simulink model "radar2jammer_god"  (R2024a)
settings: Solver=VariableStepAuto  StartTime=0.0  StopTime=inf  RelTol=1e-3
libraries: robotlib x6
settings Model: PacingRate=0.890000  Creator=bitdol  LastModifiedBy=user

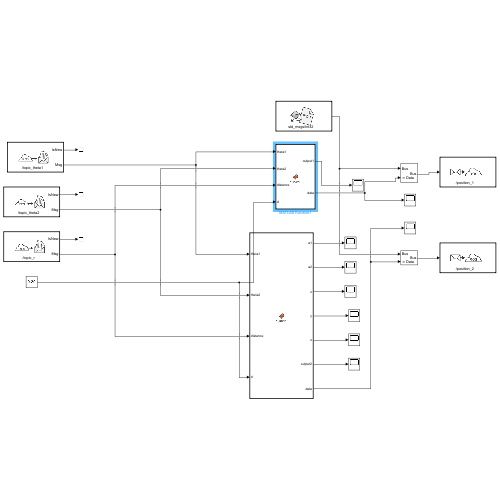
[thumbnail: Simulink's stored preview of the top-level diagram]
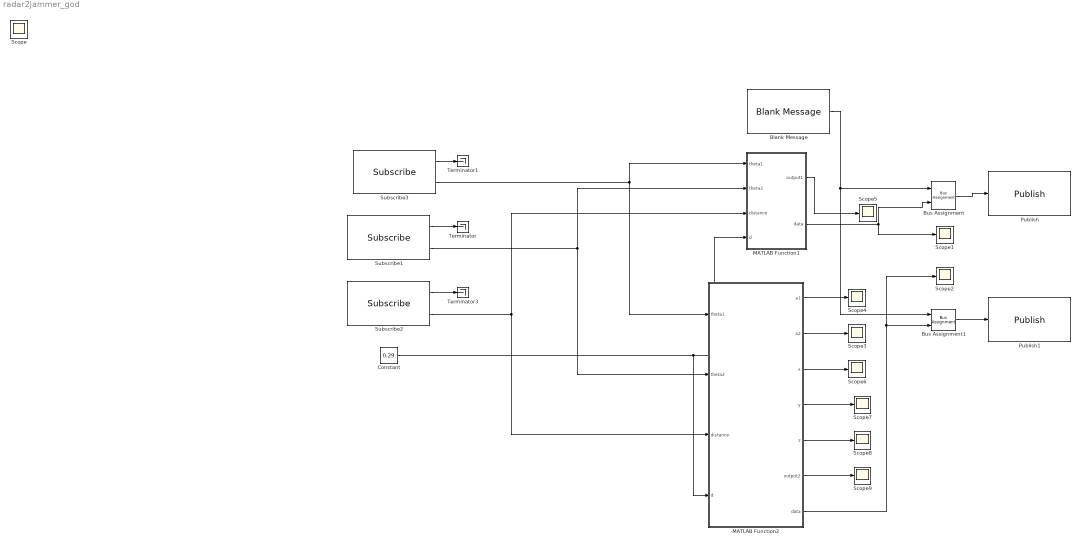
== system radar2jammer_god ==
  Blank Message : robotlib/Blank Message  messageClass=Message  entityType=std_msgs/Int32  messageType=std_msgs/Int32  SampleTime=inf  legacyBusStruct=off
  Bus Assignment : BusAssignment  AssignedSignals=Data
  Bus Assignment1 : BusAssignment  AssignedSignals=Data
  Constant : Constant  Value=0.29
  MATLAB Function1 : MATLAB Function  TreatAsAtomicUnit=on
  MATLAB Function2 : MATLAB Function  TreatAsAtomicUnit=on
  Publish : robotlib/Publish  topicSource=Specify your own  topic=/position_1  messageType=std_msgs/Int32  legacyBusStruct=off  messageQueueLength=1
  Publish1 : robotlib/Publish  topicSource=Specify your own  topic=/position_2  messageType=std_msgs/Int32  legacyBusStruct=off  messageQueueLength=1
  Scope{,1..9} (10 alike) : Scope
  Subscribe1 : robotlib/Subscribe  topicSource=Select from ROS network  topic=/topic_theta2  messageType=std_msgs/Int32  SampleTime=-1  legacyBusStruct=off  messageQueueLength=1
  Subscribe2 : robotlib/Subscribe  topicSource=Select from ROS network  topic=/topic_r  messageType=std_msgs/Int32  SampleTime=-1  legacyBusStruct=off  messageQueueLength=1
  Subscribe3 : robotlib/Subscribe  topicSource=Select from ROS network  topic=/topic_theta1  messageType=std_msgs/Int32  SampleTime=-1  legacyBusStruct=off  messageQueueLength=1
  Terminator : Terminator
  Terminator1 : Terminator
  Terminator3 : Terminator
  wires:
  Subscribe2/1 -> Terminator3/1
  Subscribe3/1 -> Terminator1/1
  Bus Assignment1/1 -> Publish1/1
  MATLAB Function2/7(data) -> Scope2/1, Bus Assignment1/2
  Subscribe1/1 -> Terminator/1
  Subscribe1/2 -> MATLAB Function1/2(theta2), MATLAB Function2/2(theta2)
  MATLAB Function1/2(data) -> Bus Assignment/2, Scope1/1
  Constant/1 -> MATLAB Function1/4(d), MATLAB Function2/4(d)
  Bus Assignment/1 -> Publish/1
  Blank Message/1 -> Bus Assignment1/1, Bus Assignment/1
  Subscribe3/2 -> MATLAB Function1/1(theta1), MATLAB Function2/1(theta1)
  Subscribe2/2 -> MATLAB Function1/3(distance), MATLAB Function2/3(distance)
  MATLAB Function1/1(output1) -> Scope5/1
  MATLAB Function2/6(output2) -> Scope9/1
  MATLAB Function2/5(z) -> Scope8/1
  MATLAB Function2/4(y) -> Scope7/1
  MATLAB Function2/3(x) -> Scope6/1
  MATLAB Function2/2(a2) -> Scope3/1
  MATLAB Function2/1(a1) -> Scope4/1

== matlab function radar2jammer_god/MATLAB Function1 ==
  data: output1 output; theta1 input; data output; theta2 input; distance input; d input
function [output1,data] = func1(theta1, theta2, distance, d)
    a1 = double((theta1.Data - 197) * (180 / 2048));
    a2 = double((theta2.Data) * (180 / 2048));
    r = double(distance.Data);
    x = (r-0.07) * cosd(a2) * cosd(a1);
    y = (r-0.07) * cosd(a2) * sind(a1);
    output1 = abs(atan2d((y+d), x)+25);

    data = int32((output1) * (2048 / 180));

== matlab function radar2jammer_god/MATLAB Function2 ==
  data: a1 output; a2 output; x output; y output; z output; output2 output; theta1 input; theta2 input; distance input; data output; d input
function [a1,a2,x,y,z,output2,data] = func2(theta1, theta2, distance, d)
    a1 = double((theta1.Data - 197) * (180 / 2048));
    a2 = double((theta2.Data ) * (180 / 2048));
    r = double(distance.Data);

    x = (r-0.07) * cosd(a2) * cosd(a1);
    y = (r-0.07) * cosd(a2) * sind(a1);
    z = (r-0.07) * sind(a2);

    output2 = abs(atan2d(z , sqrt(x^2 + (y+d)^2))-145);

    data = int32(output2*2048/180);
end
